simulink model "zad8"  (R2014b)
settings: Solver=ode45  StartTime=0.0  StopTime=70  RelTol=1e-3
values from neighbouring files (symbols this model uses):
  a1 = -0.28    [set_params.m]
  a2 = -0.9    [set_params.m]
  a3 = 0.35    [set_params.m]
  a4 = 0.3    [set_params.m]
  K = 4.5    [set_params.m]
  T1 = 5    [set_params.m]
  T2 = 8    [set_params.m]
  Tp = 1    [zad10.m]    (also in zad11.m; zad3.m = Tp_vect(i); zad9.m)
  u_lin = 1    [zad10.m]    (also in zad11.m = linspace(-1,1,101); zad12.m; zad6.m = K*a1*u + K*(a2*(u_p^2) + a3*(u_p^3) + a4*(u_p^4)) + K*(u - u; zad9.m = pkt_lin(i))
settings Model: Creator=kuba  LastModifiedBy=kuba

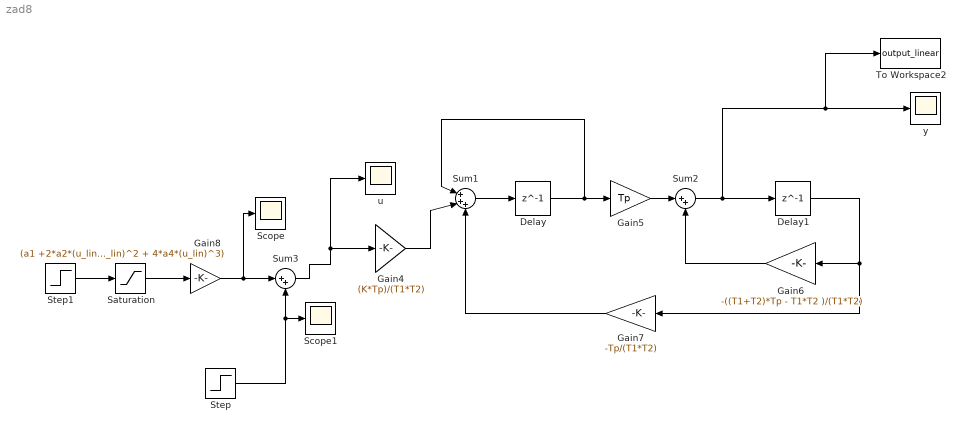
== system zad8 ==
  Delay : Delay  DelayLength=1  SampleTime=Tp
  Delay1 : Delay  DelayLength=1  SampleTime=Tp
  Gain4 : Gain  Gain=(K*Tp)/(T1*T2)
  Gain5 : Gain  Gain=Tp
  Gain6 : Gain  Gain=-((T1+T2)*Tp - T1*T2 )/(T1*T2)
  Gain7 : Gain  Gain=-Tp/(T1*T2)
  Gain8 : Gain  Gain=(a1 +2*a2*(u_lin) + 3*a3*(u_lin)^2 + 4*a4*(u_lin)^3)  SampleTime=Tp
  Saturation : Saturate  UpperLimit=1  LowerLimit=-1
  Scope : Scope
      settings: SaveName=ScopeData4
  Scope1 : Scope
      settings: SaveName=ScopeData5
  Step : Step  After=-a2*u_lin -2*a3*(u_lin^2) - 3*a4*(u_lin^3)  SampleTime=0
  Step1 : Step  SampleTime=0
  Sum1 : Sum  Inputs=|+++
  Sum2 : Sum  Inputs=|++
  Sum3 : Sum  Inputs=|++
  To Workspace2 : ToWorkspace  VariableName=output_linear  SaveFormat=Timeseries  SampleTime=-1
  u : Scope
  y : Scope
      settings: TimeRange=60  YMin=-2.5  YMax=0
  wires:
  Gain5/1 -> Sum2/1
  Gain4/1 -> Sum1/2
  Gain6/1 -> Sum2/2
  Gain7/1 -> Sum1/3
  Delay1/1 -> Gain7/1, Gain6/1
  Delay/1 -> Gain5/1, Sum1/1
  Sum2/1 -> To Workspace2/1, y/1, Delay1/1
  Sum1/1 -> Delay/1
  Sum3/1 -> u/1, Gain4/1
  Saturation/1 -> Gain8/1
  Gain8/1 -> Scope/1, Sum3/1
  Step/1 -> Scope1/1, Sum3/2
  Step1/1 -> Saturation/1
